simulink model "Kalman_State_Estimation"  (R2015a)
settings: Solver=ode45  SolverMode=SingleTasking  StartTime=0.0  StopTime=10.0  RelTol=1e-3
undefined symbols (not defined in the file or in its folder): Discrete, Time
libraries: simulink x2, ctrlSharedLib x1
settings Model: CovMetricSettings=dwe  CovHtmlReporting=off  covSaveCumulativeToWorkspaceVar=off  CovSaveSingleToWorkspaceVar=off  CovExternalEMLEnable=on  Creator=karanverma  LastModifiedBy=karanverma
settings DataIOCC: LimitDataPoints=off  SaveFormat=Dataset
settings DebuggingCC: SFUnexpectedBacktrackingDiag=error  SFNoUnconditionalDefaultTransitionDiag=error
settings HardwareCC: ProdBitPerPointer=64  ProdLargestAtomicFloat=Float  ProdIntDivRoundTo=Zero  ProdEndianess=LittleEndian  ProdHWDeviceType=Specified
settings ModelReferenceCC: PropagateSignalLabelsOutOfModel=on
settings GRTTargetCC: TargetLangStandard=C99 (ISO)  GeneratePreprocessorConditionals=Use local settings

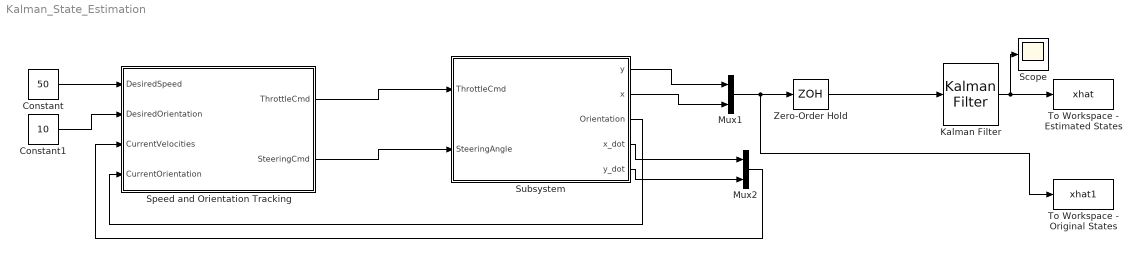
== system Kalman_State_Estimation ==
  Constant : Constant  Value=50
  Constant1 : Constant  Value=10
  Kalman Filter : ctrlSharedLib/Kalman Filter  TimeDomain=Discrete-Time  UseCurrentEstimator=on  ModelSource=Individual A, B, C, D matrices  ModelSourceVariable=ss(0.95,1,1,0,1)  A=[0 1 1;1 0 1;0 1 0]  B=1  C=[1 0 0; 0 0 1]  D=0  NumberOfStates=1  NumberOfInputs=1  NumberOfOutputs=1  InitialEstimateSource=Dialog  X0=0  P0=10  UseK=off  UseGH=off  NumberOfProcessNoiseInputs=1  G=1  TimeInvariantG=on  H=0  TimeInvariantH=on  Q=0.05  TimeInvariantQ=on  R=1  TimeInvariantR=on  N=0  TimeInvariantN=on  AddInputPort=off  AddEnablePort=off  OutputEstimatedY=off  OutputP=off  Ts=-1
  Mux1 : Mux  Inputs=2
  Mux2 : Mux  Inputs=2
  Scope : Scope
      settings: TimeRange=auto  MaxDataPoints=5000  SaveToWorkspace=off  SaveName=ScopeData  YMin=-1.46376  YMax=13.1738  SampleTime=-1
  "Speed and Orientation Tracking " : Subsystem
  Subsystem : Subsystem
  To Workspace - Estimated States : ToWorkspace  VariableName=xhat  SampleTime=-1
      settings: Save2DSignal=2-D array (concatenate along first dimension)
  "To Workspace - Original States " : ToWorkspace  VariableName=xhat1  SampleTime=-1
      settings: Save2DSignal=2-D array (concatenate along first dimension)
  Zero-Order Hold : ZeroOrderHold
  wires:
  "Speed and Orientation Tracking "/1(ThrottleCmd) -> Subsystem/1(ThrottleCmd)
  "Speed and Orientation Tracking "/2(SteeringCmd) -> Subsystem/2(SteeringAngle)
  Subsystem/3("Orientation ") -> "Speed and Orientation Tracking "/4(CurrentOrientation)
  Subsystem/4("x_dot ") -> Mux2/1
  Subsystem/5(y_dot) -> Mux2/2
  Mux2/1 -> "Speed and Orientation Tracking "/3(CurrentVelocities)
  Subsystem/2(x) -> Mux1/2
  Subsystem/1(y) -> Mux1/1
  Mux1/1 -> "To Workspace - Original States "/1, Zero-Order Hold/1
  Zero-Order Hold/1 -> Kalman Filter/1
  Kalman Filter/1 -> Scope/1, To Workspace - Estimated States/1
  Constant/1 -> "Speed and Orientation Tracking "/1(DesiredSpeed)
  Constant1/1 -> "Speed and Orientation Tracking "/2(DesiredOrientation)

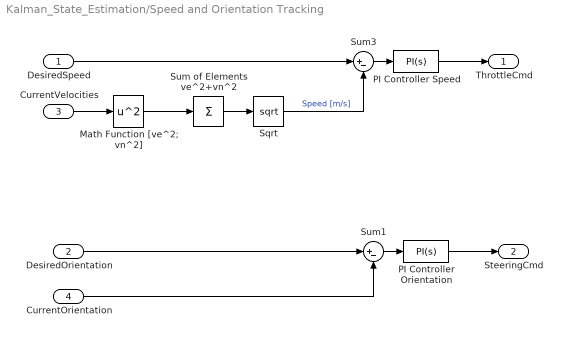
== system Kalman_State_Estimation/Speed and Orientation Tracking  ==
  DesiredSpeed : Inport
  DesiredOrientation : Inport  Port=2
  CurrentVelocities : Inport  Port=3
  CurrentOrientation : Inport  Port=4
  Math Function [ve^2; vn^2] : Math  Operator=square  SaturateOnIntegerOverflow=on
  PI Controller Orientation : simulink/Continuous/PID Controller  Controller=PI  TimeDomain=Continuous-time  SampleTime=-1  IntegratorMethod=Forward Euler  FilterMethod=Forward Euler  Form=Parallel  UseFilter=on  ControllerParametersSource=internal  P=1  I=0.3  D=0  N=100  InitialConditionSource=internal  InitialConditionForIntegrator=0  InitialConditionForFilter=0  ExternalReset=none  LimitOutput=on  UpperSaturationLimit=20  LowerSaturationLimit=-20  LinearizeAsGain=off  AntiWindupMode=clamping  Kb=1  TrackingMode=off  Kt=1  PParamMin=[]  PParamMax=[]  IParamMin=[]  IParamMax=[]  DParamMin=[]  DParamMax=[]  NParamMin=[]  NParamMax=[]  KbParamMin=[]  KbParamMax=[]  KtParamMin=[]  KtParamMax=[]  POutMin=[]  POutMax=[]  IOutMin=[]  IOutMax=[]  DOutMin=[]  DOutMax=[]  NOutMin=[]  NOutMax=[]  KbOutMin=[]  KbOutMax=[]  KtOutMin=[]  KtOutMax=[]  IntegratorOutMin=[]  IntegratorOutMax=[]  FilterOutMin=[]  FilterOutMax=[]  SumOutMin=[]  SumOutMax=[]  SumI1OutMin=[]  SumI1OutMax=[]  SumI2OutMin=[]  SumI2OutMax=[]  SumI3OutMin=[]  SumI3OutMax=[]  SumDOutMin=[]  SumDOutMax=[]  SaturationOutMin=[]  SaturationOutMax=[]  IntegratorContinuousStateAttributes=''  IntegratorStateMustResolveToSignalObject=off  IntegratorRTWStateStorageClass=Auto  FilterContinuousStateAttributes=''  FilterStateMustResolveToSignalObject=off  FilterRTWStateStorageClass=Auto  DifferentiatorICPrevScaledInput=0  DifferentiatorOutMin=[]  DifferentiatorOutMax=[]
  PI Controller Speed : simulink/Continuous/PID Controller  Controller=PI  TimeDomain=Continuous-time  SampleTime=-1  IntegratorMethod=Forward Euler  FilterMethod=Forward Euler  Form=Parallel  UseFilter=on  ControllerParametersSource=internal  P=0.15  I=0.01  D=0  N=100  InitialConditionSource=internal  InitialConditionForIntegrator=0  InitialConditionForFilter=0  ExternalReset=none  LimitOutput=on  UpperSaturationLimit=1  LowerSaturationLimit=-1  LinearizeAsGain=off  AntiWindupMode=clamping  Kb=1  TrackingMode=off  Kt=1  PParamMin=[]  PParamMax=[]  IParamMin=[]  IParamMax=[]  DParamMin=[]  DParamMax=[]  NParamMin=[]  NParamMax=[]  KbParamMin=[]  KbParamMax=[]  KtParamMin=[]  KtParamMax=[]  POutMin=[]  POutMax=[]  IOutMin=[]  IOutMax=[]  DOutMin=[]  DOutMax=[]  NOutMin=[]  NOutMax=[]  KbOutMin=[]  KbOutMax=[]  KtOutMin=[]  KtOutMax=[]  IntegratorOutMin=[]  IntegratorOutMax=[]  FilterOutMin=[]  FilterOutMax=[]  SumOutMin=[]  SumOutMax=[]  SumI1OutMin=[]  SumI1OutMax=[]  SumI2OutMin=[]  SumI2OutMax=[]  SumI3OutMin=[]  SumI3OutMax=[]  SumDOutMin=[]  SumDOutMax=[]  SaturationOutMin=[]  SaturationOutMax=[]  IntegratorContinuousStateAttributes=''  IntegratorStateMustResolveToSignalObject=off  IntegratorRTWStateStorageClass=Auto  FilterContinuousStateAttributes=''  FilterStateMustResolveToSignalObject=off  FilterRTWStateStorageClass=Auto  DifferentiatorICPrevScaledInput=0  DifferentiatorOutMin=[]  DifferentiatorOutMax=[]
  Sqrt : Sqrt  SaturateOnIntegerOverflow=on
  Sum of Elements ve^2+vn^2 : Sum  Inputs=+
  Sum1 : Sum  Inputs=|+-
  Sum3 : Sum  Inputs=|+-
  ThrottleCmd : Outport
  SteeringCmd : Outport  Port=2
  wires:
  PI Controller Speed/1 -> ThrottleCmd/1
  DesiredSpeed/1 -> Sum3/1
  Sum3/1 -> PI Controller Speed/1
  Math Function [ve^2; vn^2]/1 -> Sum of Elements ve^2+vn^2/1
  CurrentVelocities/1 -> Math Function [ve^2; vn^2]/1
  Sum of Elements ve^2+vn^2/1 -> Sqrt/1
  Sqrt/1 -> Sum3/2  "Speed [m/s]"
  DesiredOrientation/1 -> Sum1/1
  PI Controller Orientation/1 -> SteeringCmd/1
  Sum1/1 -> PI Controller Orientation/1
  CurrentOrientation/1 -> Sum1/2

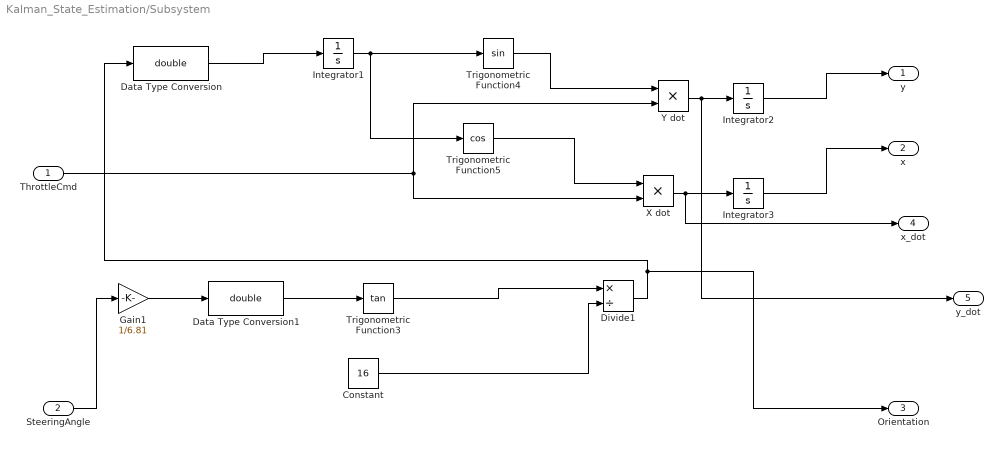
== system Kalman_State_Estimation/Subsystem ==
  ThrottleCmd : Inport
  SteeringAngle : Inport  Port=2
  Constant : Constant  Value=16
  Data Type Conversion : DataTypeConversion  OutDataTypeStr=double
  Data Type Conversion1 : DataTypeConversion  OutDataTypeStr=double
  Divide1 : Product  Inputs=*/
  Gain1 : Gain  Gain=1/6.81
  Integrator1 : Integrator
  Integrator2 : Integrator
  Integrator3 : Integrator
  Trigonometric Function3 : Trigonometry  Operator=tan  OutputSignalType=real
  Trigonometric Function4 : Trigonometry
  Trigonometric Function5 : Trigonometry  Operator=cos
  "X dot " : Product
  "Y dot " : Product
  y : Outport
  x : Outport  Port=2
  "Orientation " : Outport  Port=3
  "x_dot " : Outport  Port=4
  y_dot : Outport  Port=5
  wires:
  Gain1/1 -> Data Type Conversion1/1
  Integrator1/1 -> Trigonometric Function5/1, Trigonometric Function4/1
  ThrottleCmd/1 -> "X dot "/2, "Y dot "/2
  Trigonometric Function5/1 -> "X dot "/1
  Trigonometric Function4/1 -> "Y dot "/1
  "X dot "/1 -> "x_dot "/1, Integrator3/1
  "Y dot "/1 -> y_dot/1, Integrator2/1
  Data Type Conversion/1 -> Integrator1/1
  Integrator2/1 -> y/1
  Integrator3/1 -> x/1
  SteeringAngle/1 -> Gain1/1
  Data Type Conversion1/1 -> Trigonometric Function3/1
  Trigonometric Function3/1 -> Divide1/1
  Constant/1 -> Divide1/2
  Divide1/1 -> "Orientation "/1, Data Type Conversion/1
